simulink model "s0431"  (Simulink 7.0)
settings: Solver=ode3  SolverMode=SingleTasking  StartTime=0.0  StopTime=10  FixedStep=1  MaxStep=1  RelTol=1e-3  AbsTol=1e-6
values from neighbouring files (symbols this model uses):
  Gsnen = Gs.den{1}    [m0404Bsp.m]
  Gszae = Gs.num{1}    [m0404Bsp.m]
  Tt = .4    (= 0.4)    [m0108d.m]    (also in m0259.m = 1; m0314.m = 2.13; m0322.m = 0.8; m0326.m = 4)
  w_steptime = w_steptime-t0A    (= 6)    [m0404Bsp.m]
  wdach_ = wdach    (= 1)    [m0404Bsp.m]
  z_steptime = z_steptime-t0A    (= 1)    [m0404Bsp.m]
  zdach_ = zdach    (= 1)    [m0404Bsp.m]
undefined symbols (not defined in the file or in its folder): xD, zdach0
libraries: simulink x1
settings Model: Creator=froriep  LastModifiedBy=froriep
settings DataIOCC: LimitDataPoints=off  SaveOutput=off  SaveTime=off
settings OptimizationCC: BooleanDataType=off
settings DebuggingCC: SaveWithParameterizedLinksMsg=none  SignalResolutionControl=TryResolveAllWithWarning  SolverPrmCheckMsg=none  MultiTaskDSMMsg=warning  MultiTaskCondExecSysMsg=none  StrictBusMsg=None
settings HardwareCC: TargetUnknown=on
settings RTWCC: IncludeERTFirstTime=on

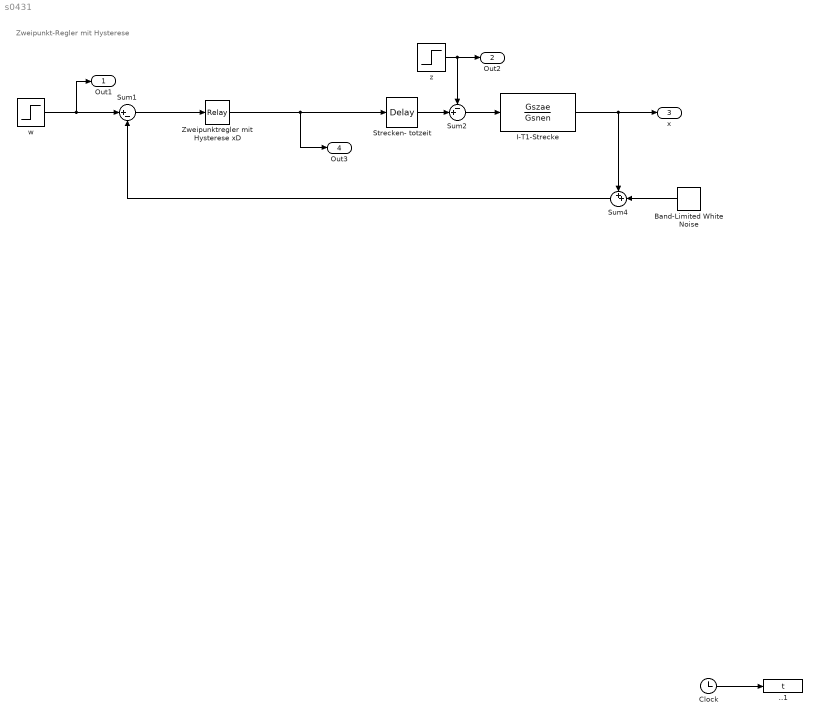
== system s0431 ==
  note: Zweipunkt-Regler mit Hysterese
  ..1 : ToWorkspace  VariableName=t  SaveFormat=Array
  Band-Limited White Noise : simulink/Sources/Band-Limited White Noise  Orientation=left  SystemSampleTime=-1  Cov=Rauschen  Ts=.01  seed=[23341]
  Clock : Clock
      settings: Decimation=10
  I-T1-Strecke : TransferFcn  Numerator=Gszae  Denominator=Gsnen
  Strecken- totzeit : TransportDelay  DelayTime=Tt
  Sum1 : Sum  Inputs=|+-  SaturateOnIntegerOverflow=on  InputSameDT=on
  Sum2 : Sum  Inputs=-+|  SaturateOnIntegerOverflow=on  InputSameDT=on
  Sum4 : Sum  Orientation=left  Inputs=++|  SaturateOnIntegerOverflow=on  InputSameDT=on
  Zweipunktregler mit Hysterese xD : Relay  OnSwitchValue=xD/2  OffSwitchValue=-xD/2  OnOutputValue=Yh  OutDataType=sfix(16)  OutScaling=2^0
  w : Step  Time=w_steptime  After=wdach_  SampleTime=0
  z : Step  Time=z_steptime  After=zdach0+zdach_  SampleTime=0
  Out1 : Outport  OutDataType=sfix(16)  OutScaling=2^0
  Out2 : Outport  Port=2  OutDataType=sfix(16)  OutScaling=2^0
  x : Outport  Port=3  OutDataType=sfix(16)  OutScaling=2^0
  Out3 : Outport  Port=4  OutDataType=sfix(16)  OutScaling=2^0
  wires:
  z/1 -> Sum2/1, Out2/1
  w/1 -> Sum1/1, Out1/1
  Clock/1 -> ..1/1
  I-T1-Strecke/1 -> x/1, Sum4/1
  Sum4/1 -> Sum1/2
  Band-Limited White Noise/1 -> Sum4/2
  Sum1/1 -> Zweipunktregler mit Hysterese xD/1
  Zweipunktregler mit Hysterese xD/1 -> Out3/1, Strecken- totzeit/1
  Strecken- totzeit/1 -> Sum2/2
  Sum2/1 -> I-T1-Strecke/1
